simulink model "Part3"  (R2024b)
settings: Solver=VariableStepAuto  StartTime=0.0  StopTime=tspan  FixedStep=10  RelTol=1e-8
model workspace (MATLAB code in the model file):
  | mu = 398601; % km
  | Re = 6378.137; %km
values from neighbouring files (symbols this model uses):
  Eul0_b_eci = Eul0_b_eci(:)    [Final_3.m]    (also in ORR_part4_script.m = [phi_b_eci_0; theta_b_eci_0; psi_b_eci_0]; Part2_TorqueFreeMotion.m = [phi_b_eci_0; theta_b_eci_0; psi_b_eci_0]; Part2_TorqueFreeMotion_SS.m = [phi_b_eci_0; theta_b_eci_0; psi_b_eci_0]; Part5_TorqueFreeMotion_SS.m = [phi_b_eci_0; theta_b_eci_0; psi_b_eci_0])
  J = n.sat.I    [Part5_TorqueFreeMotion_SS.m]    (also in Part_2_TorqueFreeMotion_Orr.m = [812.0396         0         0; Part_5_ORR.m = [d.Ixx, d.Ixy, d.Ixz;         d.Ixy, d.Iyy, d.Iyz;         d)
  JD_0 = 2460390    [Final_3.m]    (also in ORR_part4_script.m; Part3_Disturbance.m; Part_3_Disturbance_ORR.m)
  m_b = [0; 0; -0.5]    [Final_3.m]    (also in ORR_part4_script.m)
  q0_b_eci = q0_b_eci(:)    [Final_3.m]    (also in ORR_part4_script.m; Part2_TorqueFreeMotion.m = DCM_to_quat(C_b_ECI_0); Part2_TorqueFreeMotion_SS.m = DCM_to_quat(C_b_ECI_0); Part5_TorqueFreeMotion_SS.m = DCM_to_quat(C_b_ECI_0))
  r_ECI_0 = r0eci_vec    [Final_3.m]    (also in ORR_part4_script.m)
  sun_ECI = [1; 0; 0]    [Final_3.m]    (also in ORR_part4_script.m)
  surfaceProperties = [n.sat.areas n.sat.rho n.sat.normal]    [Final_3.m]    (also in ORR_part4_script.m; Part_3_Disturbance_ORR.m = [Areas cps normals])
  T_c = [0; 0; 0]    [Final_3.m]    (also in Final_4.m; ORR_part4_script.m; Part3_Disturbance.m; Part_3_Disturbance_ORR.m)
  v_ECI_0 = v0eci_vec    [Final_3.m]    (also in ORR_part4_script.m)
  w0_b_eci = [0.001; -0.001; 0.002]    [Part2_TorqueFreeMotion.m]    (also in Part2_TorqueFreeMotion_SS.m; Part5_TorqueFreeMotion_SS.m)
settings Model: Creator=emehiel  LastModifiedBy=dstan
settings SolverCC: AlgebraicLoopSolver=TrustRegion
settings DebuggingCC: UnconnectedInputMsg=warning  UnconnectedOutputMsg=warning  UnconnectedLineMsg=warning
settings ModelReferenceCC: EnableRefExpFcnMdlSchedulingChecks=on
settings RTWCC: GPUComputeCapability=3.5

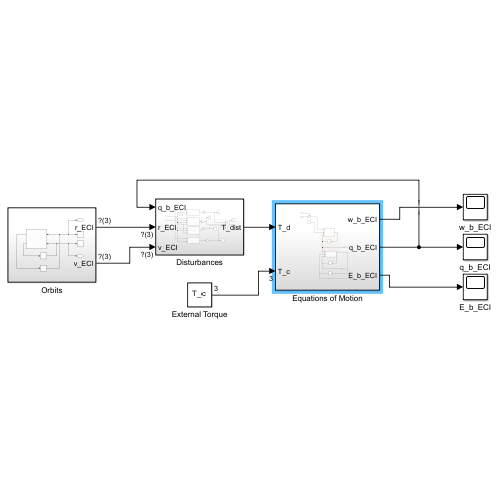
[thumbnail: Simulink's stored preview of the top-level diagram]
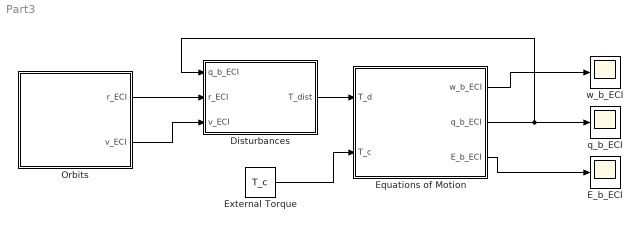
== system Part3 ==
  Disturbances : Subsystem
  E_b_ECI : Scope
  Equations of Motion : Subsystem
  External Torque : Constant  Value=T_c
  Orbits : Subsystem
  q_b_ECI : Scope
  w_b_ECI : Scope
  wires:
  Orbits/1(r_ECI) -> Disturbances/2(r_ECI)
  Orbits/2(v_ECI) -> Disturbances/3(v_ECI)
  Equations of Motion/2(q_b_ECI) -> Disturbances/1(q_b_ECI), q_b_ECI/1
  Equations of Motion/1(w_b_ECI) -> w_b_ECI/1
  Disturbances/1(T_dist) -> Equations of Motion/1(T_d)
  Equations of Motion/3(E_b_ECI) -> E_b_ECI/1
  External Torque/1 -> Equations of Motion/2(T_c)

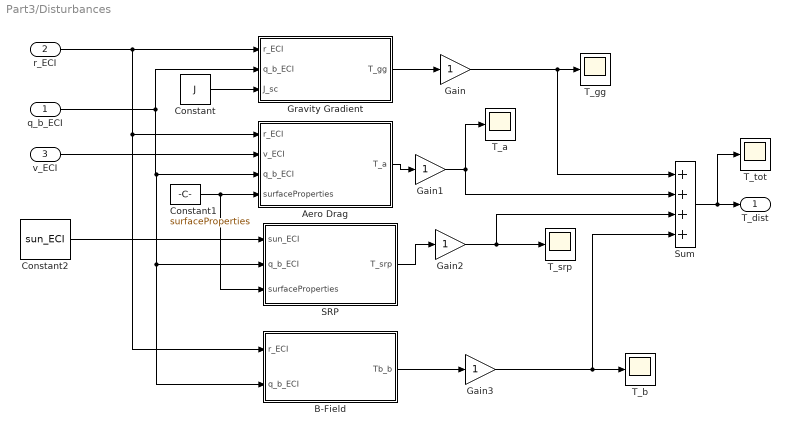
== system Part3/Disturbances ==
  q_b_ECI : Inport
  r_ECI : Inport  Port=2
  v_ECI : Inport  Port=3
  Aero Drag : MATLAB Function  TreatAsAtomicUnit=on
  B-Field : Subsystem
  Constant : Constant  Value=J
  Constant1 : Constant  Value=surfaceProperties
  Constant2 : Constant  Value=sun_ECI
  Gain{,1..3} (4 alike) : Gain
  Gravity Gradient : MATLAB Function  TreatAsAtomicUnit=on
  SRP : MATLAB Function  TreatAsAtomicUnit=on
  Sum : Sum  Inputs=++++
  T_a : Scope
  T_b : Scope
  T_gg : Scope
  T_srp : Scope
  T_tot : Scope
  T_dist : Outport
  wires:
  Sum/1 -> T_tot/1, T_dist/1
  Aero Drag/1(T_a) -> Gain1/1
  Gravity Gradient/1(T_gg) -> Gain/1
  SRP/1(T_srp) -> Gain2/1
  Constant1/1 -> SRP/3(surfaceProperties), Aero Drag/4(surfaceProperties)
  v_ECI/1 -> Aero Drag/2(v_ECI)
  q_b_ECI/1 -> B-Field/2(q_b_ECI), SRP/2(q_b_ECI), Aero Drag/3(q_b_ECI), Gravity Gradient/2(q_b_ECI)
  Constant/1 -> Gravity Gradient/3(J_sc)
  Constant2/1 -> SRP/1(sun_ECI)
  r_ECI/1 -> B-Field/1(r_ECI), Aero Drag/1(r_ECI), Gravity Gradient/1(r_ECI)
  B-Field/1(Tb_b) -> Gain3/1
  Gain/1 -> Sum/1, T_gg/1
  Gain1/1 -> Sum/2, T_a/1
  Gain2/1 -> Sum/3, T_srp/1
  Gain3/1 -> T_b/1, Sum/4

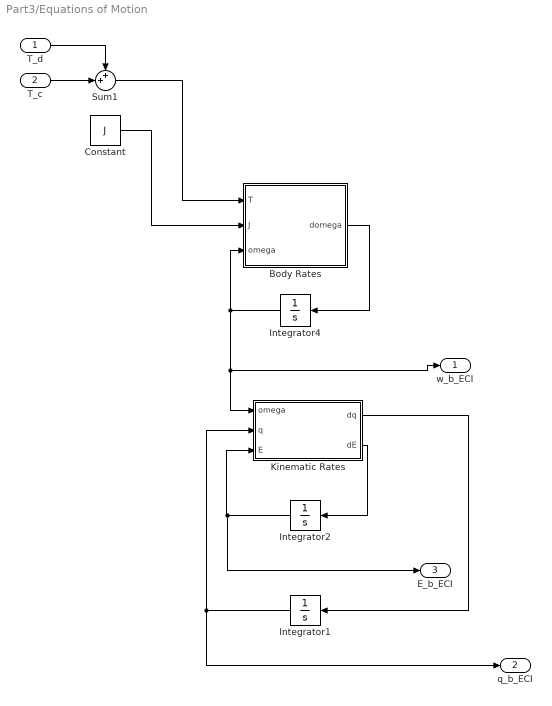
== system Part3/Equations of Motion ==
  T_d : Inport
  T_c : Inport  Port=2
  Body Rates : MATLAB Function  TreatAsAtomicUnit=on
  Constant : Constant  Value=J
  Integrator1 : Integrator  InitialCondition=q0_b_eci
  Integrator2 : Integrator  InitialCondition=Eul0_b_eci
  Integrator4 : Integrator  InitialCondition=w0_b_eci
  Kinematic Rates : MATLAB Function  TreatAsAtomicUnit=on
  Sum1 : Sum  Inputs=++|
  w_b_ECI : Outport  VectorParamsAs1DForOutWhenUnconnected=off
  q_b_ECI : Outport  Port=2  VectorParamsAs1DForOutWhenUnconnected=off
  E_b_ECI : Outport  Port=3  VectorParamsAs1DForOutWhenUnconnected=off
  wires:
  Integrator2/1 -> E_b_ECI/1, Kinematic Rates/3(E)
  T_d/1 -> Sum1/1
  T_c/1 -> Sum1/2
  Integrator1/1 -> q_b_ECI/1, Kinematic Rates/2(q)
  Integrator4/1 -> Body Rates/3(omega), w_b_ECI/1, Kinematic Rates/1(omega)
  Kinematic Rates/2(dE) -> Integrator2/1
  Body Rates/1(domega) -> Integrator4/1
  Sum1/1 -> Body Rates/1(T)
  Constant/1 -> Body Rates/2(J)
  Kinematic Rates/1(dq) -> Integrator1/1

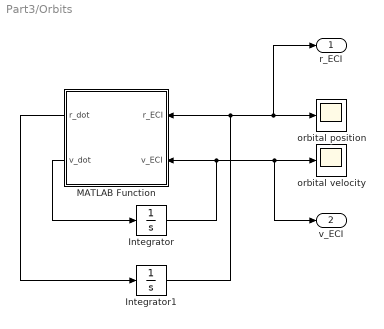
== system Part3/Orbits ==
  Integrator : Integrator  InitialCondition=v_ECI_0
  Integrator1 : Integrator  InitialCondition=r_ECI_0
  MATLAB Function : MATLAB Function  TreatAsAtomicUnit=on
  orbital position : Scope
  orbital velocity : Scope
  r_ECI : Outport  VectorParamsAs1DForOutWhenUnconnected=off
  v_ECI : Outport  Port=2  VectorParamsAs1DForOutWhenUnconnected=off
  wires:
  Integrator/1 -> v_ECI/1, orbital velocity/1, MATLAB Function/2(v_ECI)
  Integrator1/1 -> r_ECI/1, orbital position/1, MATLAB Function/1(r_ECI)
  MATLAB Function/1(r_dot) -> Integrator1/1
  MATLAB Function/2(v_dot) -> Integrator/1

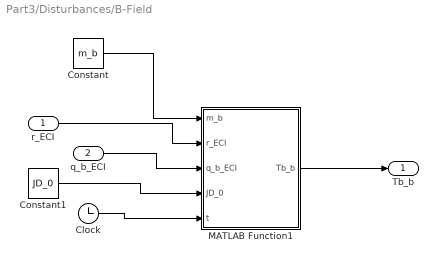
== system Part3/Disturbances/B-Field ==
  r_ECI : Inport
  q_b_ECI : Inport  Port=2
  Clock : Clock
  Constant : Constant  Value=m_b  VectorParams1D=off
  Constant1 : Constant  Value=JD_0
  MATLAB Function1 : MATLAB Function  TreatAsAtomicUnit=on
  Tb_b : Outport
  wires:
  MATLAB Function1/1(Tb_b) -> Tb_b/1
  q_b_ECI/1 -> MATLAB Function1/3(q_b_ECI)
  r_ECI/1 -> MATLAB Function1/2(r_ECI)
  Clock/1 -> MATLAB Function1/5(t)
  Constant1/1 -> MATLAB Function1/4(JD_0)
  Constant/1 -> MATLAB Function1/1(m_b)

== matlab function Part3/Equations of Motion/Body Rates ==
  data: T input; J input; omega input; domega output
function domega = dynamics(T, J, omega)

%column vecs
omega = omega(:);
T = T(:);

domega = J \ (T - cross(omega, J*omega));
end

== matlab function Part3/Equations of Motion/Kinematic Rates ==
  data: omega input; q input; dq output; E input; dE output
function [dq, dE] = kinematics(omega, q, E)
% column vecs
omega = omega(:);
q = q(:);
E = E(:);

% unpack euler angles
phi = E(1);
theta = E(2);
psi = E(3);

% unpack quat
eps = q(1:3);
eta = q(4);

% euler derivative
B = [1, sin(phi)*tan(theta),  cos(phi)*tan(theta);
     0, cos(phi),            -sin(phi);
     0, sin(phi)/cos(theta),  cos(phi)/cos(theta)];

dE = B * omega;

% quat derivative
dq = zeros(4,1);
dq(1:3) = 0.5 * ((eta*eye(3) + skew(eps)) * omega);
dq(4)   = -0.5 * (eps.' * omega);

end

== matlab function Part3/Disturbances/Gravity Gradient ==
  data: r_ECI input; T_gg output; q_b_ECI input; J_sc input
function T_gg = gg_torque(r_ECI, q_b_ECI, J_sc)
% Gravity-gradient torque in body coordinates
% Textbook model used:
%   Tg = (3*mu/r^5) * (r_b x (I*r_b))

    T_gg = zeros(3,1);

    % Earth gravitational parameter in SI [m^3/s^2]
    mu = 3.986004418e14;

    % Quaternion -> DCM, ECI to body
    q = q_b_ECI(:);
    e = q(1:3);
    eta = q(4);
    C_b_eci = (eta^2 - e.'*e)*eye(3) + 2*(e*e.') - 2*eta*vect2cross(e);

    % Convert r from km to m so units match J_sc [kg m^2]
    r_b = C_b_eci * (1000 * r_ECI(:));
    r   = norm(r_b);

    if r < 1e-12
        return
    end

    T_gg = (3 * mu / r^5) * cross(r_b, J_sc * r_b);
end

function C = vect2cross(v)
    C = [ 0    -v(3)  v(2);
          v(3)  0    -v(1);
         -v(2)  v(1)  0   ];
end

== matlab function Part3/Disturbances/Aero Drag ==
  data: r_ECI input; v_ECI input; T_a output; q_b_ECI input; surfaceProperties input
function T_a = aero_drag_torque(r_ECI, v_ECI, q_b_ECI, surfaceProperties)
T_a = zeros(3,1);
Cd = 2.5;

q   = q_b_ECI(:);
eps = q(1:3);
eta = q(4);
C_b_eci = (eta^2 - eps'*eps)*eye(3) + 2*(eps*eps') - 2*eta*vect2cross(eps);

v_b_m  = C_b_eci * v_ECI(:) * 1000;
v_mag  = norm(v_b_m);
v_unit = v_b_m / v_mag;

alt = norm(r_ECI) - 6378.137;
rho = atmospheric_density(alt);

for i = 1:size(surfaceProperties, 1)
    area   = surfaceProperties(i, 1);
    cp     = surfaceProperties(i, 2:4)';
    normal = surfaceProperties(i, 5:7)';
    A_wet  = area * dot(normal, v_unit);
    if A_wet > 0
        F   = -(1/2) * rho * v_mag^2 * Cd * A_wet * v_unit;
        T_a = T_a + cross(cp, F);
    end
end
end

function C = vect2cross(v)
C = [ 0,   -v(3),  v(2);
      v(3),  0,   -v(1);
     -v(2),  v(1),  0  ];
end

function rho = atmospheric_density(alt)
    rho = 0.0;
    h0   = [0, 25, 30, 35, 40, 45, 50, 55, 60, 65, 70, 75, 80, 85, 90, ...
            95, 100, 110, 120, 130, 140, 150, 160, 180, 200, 250, 300, ...
            350, 400, 450, 500, 600, 700, 800, 900, 1000];
    rho0 = [1.225, 3.899e-2, 1.774e-2, 8.279e-3, 3.972e-3, 1.995e-3, ...
            1.057e-3, 5.821e-4, 3.206e-4, 1.718e-4, 8.770e-5, 4.178e-5, ...
            1.905e-5, 8.337e-6, 3.396e-6, 1.343e-6, 5.297e-7, 9.661e-8, ...
            2.438e-8, 8.484e-9, 3.845e-9, 2.070e-9, 1.224e-9, 5.464e-10, ...
            2.789e-10, 7.248e-11, 2.418e-11, 9.158e-12, 3.725e-12, ...
            1.585e-12, 6.967e-13, 1.454e-13, 3.614e-14, 1.170e-14, ...
            5.245e-15, 3.019e-15];
    H    = [8.44, 6.49, 6.75, 7.07, 7.47, 7.83, 7.95, 7.73, 7.29, 6.81, ...
            6.33, 6.00, 5.70, 5.41, 5.38, 5.74, 6.15, 8.06, 11.6, 16.1, ...
            20.6, 24.6, 26.3, 33.2, 38.5, 46.9, 52.5, 56.4, 59.4, 62.2, ...
            65.8, 79.0, 109.0, 164.0, 225.0, 268.0];

    idx = 1;  % default scalar
    for k = 1:length(h0)
        if alt >= h0(k)
            idx = k;
        end
    end

    rho = rho0(idx) * exp(-(alt - h0(idx)) / H(idx));
end

== matlab function Part3/Disturbances/SRP ==
  data: sun_ECI input; T_srp output; q_b_ECI input; surfaceProperties input
function T_srp = SPR_torque(sun_ECI, q_b_ECI, surfaceProperties)
% SRP torque in body coordinates
%
% Inputs:
%   sun_ECI           3x1 sun direction in ECI
%   q_b_ECI           4x1 quaternion [eps1; eps2; eps3; eta]
%   surfaceProperties Nx7 = [area, rho_x, rho_y, rho_z, n_x, n_y, n_z]
%
% Output:
%   T_srp             3x1 SRP torque in body frame [N m]
%
% Textbook model used:
%   total absorption
%   F_i = -p * A_i * max(n_i dot s_b, 0) * s_b
%   T_i = rho_i x F_i

    T_srp = zeros(3,1);

    % Solar radiation pressure near Earth [N/m^2]
    p = 4.5e-6;

    % Quaternion -> DCM, ECI to body
    q = q_b_ECI(:);
    e = q(1:3);
    eta = q(4);
    C_b_eci = (eta^2 - e.'*e)*eye(3) + 2*(e*e.') - 2*eta*vect2cross(e);

    % Sun direction in body frame
    s_b = -C_b_eci * sun_ECI(:);
    s_norm = norm(s_b);
    

    if s_norm < 1e-12
        return
    end

    s_hat = s_b / s_norm;

    % Loop over surfaces
    for i = 1:size(surfaceProperties,1)
        area   = surfaceProperties(i,1);
        rho_i  = surfaceProperties(i,2:4).';
        n_i    = surfaceProperties(i,5:7).';

        % illuminated if n dot s >= 0
        cos_alpha = dot(n_i, s_hat);

        if cos_alpha > 0
            F_i   = -p * area * cos_alpha * s_hat;
            T_srp = T_srp + cross(rho_i, F_i);
        end
    end
end

function C = vect2cross(v)
    C = [ 0    -v(3)  v(2);
          v(3)  0    -v(1);
         -v(2)  v(1)  0   ];
end

== matlab function Part3/Orbits/MATLAB Function ==
  data: r_ECI input; r_dot output; v_ECI input; v_dot output
function [r_dot, v_dot] = orbitalDynamics(r_ECI, v_ECI)

mu = 398600.0;

r = sqrt(r_ECI(1)^2 + r_ECI(2)^2 + r_ECI(3)^2);

r_dot = [v_ECI(1); v_ECI(2); v_ECI(3)];
v_dot = -(mu / r^3) * [r_ECI(1); r_ECI(2); r_ECI(3)];

end

== matlab function Part3/Disturbances/B-Field/MATLAB Function1 ==
  data: m_b input; r_ECI input; q_b_ECI input; Tb_b output; JD_0 input; t input
function Tb_b = WMM(m_b, r_ECI, q_b_ECI, JD_0, t)

m_b = m_b(:);
r_ECI = r_ECI(:);
q_b_ECI = q_b_ECI(:);

% DGRF 2020 (given)
% a = 6371.2; %km
% g_11 = -1450.9; %nT
% h_11 = 4652.5; %nT
% g_10 = -29404.8; %nT
% m_ECEF = a^3*[g_11; h_11; g_10];

% converting given values to m and T
a = 6371.2 * 10^3;
g_11 = -1450.9 * 10^-9; 
h_11 = 4652.5 * 10^-9; 
g_10 = -29404.8 * 10^-9; 
m_ECEF = a^3*[g_11; h_11; g_10];

% local time is noon at initial given state, assuming t is in seconds
JD = JD_0 + t / 86400;

% first convert r from eci to ecef 

C_ecef_eci = eci2ecef(JD);

r_ECEF = C_ecef_eci * (1000 * r_ECI);

r = norm(r_ECEF);

B_ecef = (3 * (m_ECEF.' * r_ECEF) * r_ECEF - r^2 * m_ECEF) / r^5;

C_b_ECI = quat2C(q_b_ECI);

C_b_ecef = C_b_ECI * C_ecef_eci'; % doing successive rotions and transposing to get C_b_eci * C_eci_ecef

B_b = C_b_ecef * B_ecef;

Tb_b = vcross(m_b) * B_b;



    function C_ecef_eci = eci2ecef(JD) 
        T0 = (JD - 2451545) / 36525; 
        theta_G = mod(100.4606184 + 36000.77004*T0 + 0.000387933*T0^2 - 2.58*10^-8 * T0^3, 360); % in degs 
        theta_G = deg2rad(theta_G);
    
        C_ecef_eci = [cos(theta_G) sin(theta_G) 0
            -sin(theta_G) cos(theta_G) 0
            0 0 1]; % negative rotation about z axis 

    end 

        function vCross = vcross(v)
            vCross = [ 0,    -v(3),  v(2)
                      v(3),    0,   -v(1)
                     -v(2),   v(1),   0];
        end
        

        function C21 = quat2C(quaternion)
           
            epsilon = quaternion(1:3);
            eta = quaternion(4);
            I = [1 0 0
                0 1 0
                0 0 1];
            C21 = (2 * eta^2 - 1) * I + 2 * (epsilon * epsilon') - 2 * eta * vcross(epsilon);

        
        end

end
